simulink model "robot_diff_flatness"  (R2015b)
settings: Solver=FixedStepAuto  StartTime=0.0  StopTime=P.T  RelTol=1e-3
InitFcn:
  | param
undefined symbols (not defined in the file or in its folder): ctrl, drawEnvironment, P
settings Model: Creator=beard  LastModifiedBy=magiccjae
settings DataIOCC: SaveFormat=Array
settings DebuggingCC: UnderspecifiedInitializationDetection=Classic  MergeDetectMultiDrivingBlocksExec=none  SolverPrmCheckMsg=warning  StateNameClashWarn=warning
settings HardwareCC: ProdBitPerPointer=32  ProdLargestAtomicFloat=None  ProdIntDivRoundTo=Undefined  ProdEndianess=Unspecified  ProdWordSize=32  ProdHWDeviceType=32-bit Generic
settings GRTTargetCC: GeneratePreprocessorConditionals=Disable all
settings ConfigComp: CovModelRefEnable=Off

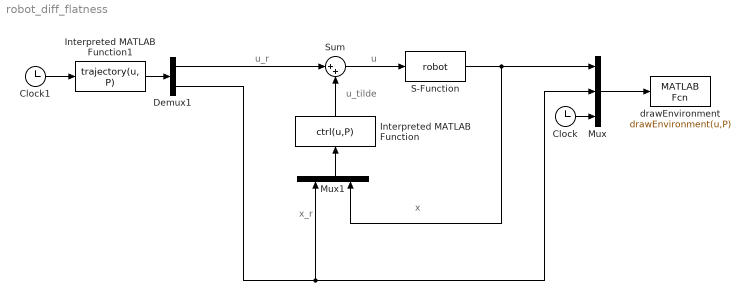
== system robot_diff_flatness ==
  note: x
  note: x_r
  note: u
  note: u_tilde
  note: u_r
  Clock : Clock
  Clock1 : Clock
  Demux1 : Demux  Outputs=[2 6]
  Interpreted MATLAB Function : MATLABFcn  MATLABFcn=ctrl(u,P)  OutputDimensions=2  SampleTime=.01
  Interpreted MATLAB Function1 : MATLABFcn  MATLABFcn=trajectory(u, P)  OutputDimensions=8
  Mux : Mux  Inputs=3
  Mux1 : Mux  Inputs=2
  S-Function : S-Function  FunctionName=robot  Parameters=P  SFunctionDeploymentMode=off  EnableBusSupport=off
  Sum : Sum  Inputs=|++
  drawEnvironment : MATLABFcn  MATLABFcn=drawEnvironment(u,P)  OutputDimensions=0
  wires:
  Clock/1 -> Mux/3
  S-Function/1 -> Mux1/2, Mux/1
  Mux/1 -> drawEnvironment/1
  Demux1/2 -> Mux/2, Mux1/1
  Sum/1 -> S-Function/1
  Demux1/1 -> Sum/1
  Interpreted MATLAB Function/1 -> Sum/2
  Mux1/1 -> Interpreted MATLAB Function/1
  Clock1/1 -> Interpreted MATLAB Function1/1
  Interpreted MATLAB Function1/1 -> Demux1/1
